simulink model "Overtaking"  (R2024a)
settings: Solver=FixedStepDiscrete  StartTime=0.0  StopTime=inf  FixedStep=0.001  RelTol=1e-3  EnableMultiTasking=on
undefined symbols (not defined in the file): route1_frenet, route1_waypoint, route2_frenet, route2_waypoint, route3_frenet, route3_waypoint, route4_frenet, route4_waypoint, route5_frenet, route5_waypoint
libraries: CarMaker4SL x49, simulink x1
(part 4 of 4)

== matlab function Overtaking/CarMaker/Subsystem/Final Project/Scenario 1/Waypoint_Follower1 ==
  settings: sampleTime=0.1
  data: local_waypoints input; steering_angle output; state input; change_dist input; target_idx output
% local tracking
function [steering_angle, target_idx] = waypoint_follower(local_waypoints, state, change_dist)

    WHEEL_BASE = 2.9;
    lookahead_dist = 6.0;
    
    % % sigmoid lookahead_dist change
    % if(change_dist > 1.8) 
    %     lookahead_dist = (10 / (1 + exp(-0.4 * change_dist))) + 5;
    % end
    % 
    % % final state -> parking area entry
    % if(state == 7)
    %     lookahead_dist = 2.5;
    % end

    target_idx = -1;
    final_ld = 0;

    for i = 1:size(local_waypoints, 1)
        dist = norm(local_waypoints(i, :));
        if dist > lookahead_dist && local_waypoints(i, 1) > 0
            target_idx = i;
            final_ld = dist;
            break;
        end
    end

    if target_idx == -1
        steering_angle = 0;
        return;
    end

    target_point = local_waypoints(target_idx, :);
    alpha = atan2(target_point(2), target_point(1));
    alpha = wrapToPi(alpha);

    final_ld = min(max(final_ld, 2.0), 20.0); 

    steering_angle = atan2(2 * WHEEL_BASE * sin(alpha), final_ld);
end


% % global tracking
% function [steering_angle, start_idx] = pure_pursuit(waypoints, vehicle_position, head)
% 
%     persistent last_target_idx;
%     if isempty(last_target_idx)
%         last_target_idx = 1; % 초기값 설정
%     end
% 
%     WHEEL_BASE = 2.7;
% 
%     waypoints_x = waypoints(:,1);
%     waypoints_y = waypoints(:,2);
%     % num_points = length(waypoints_x);
%     num_points = 300;
% 
%     local_waypoints = zeros(num_points, 2);
%     x_ego = vehicle_position(1);
%     y_ego = vehicle_position(2);
% 
%     for i = 1:num_points
%         dx = waypoints_x(i) - x_ego;
%         dy = waypoints_y(i) - y_ego;
% 
%         local_x = dx * cos(-head) - dy * sin(-head);
%         local_y = dx * sin(-head) + dy * cos(-head);
% 
%         local_waypoints(i, :) = [local_x, local_y];
%     end    
% 
%     lookahead_dist = 5.0;
% 
%     distances_to_waypoints = sqrt((waypoints_x - x_ego).^2 + (waypoints_y - y_ego).^2);
%     [~, closest_idx] = min(distances_to_waypoints);
% 
%     start_idx = max(last_target_idx, closest_idx);
% 
%     target_idx = -1;
%     final_ld = 0;
%     for i = start_idx:num_points
%         dist = norm(local_waypoints(i, :));
%         if dist > lookahead_dist && local_waypoints(i, 1) > 0
%             target_idx = i;
%             final_ld = dist;
%             break;
%         end
%     end
% 
%     if target_idx == -1
%         for i = 1:start_idx-1
%             dist = norm(local_waypoints(i, :));
%             if dist > lookahead_dist && local_waypoints(i, 1) > 0
%                 target_idx = i;
%                 final_ld = dist;
%                 break;
%             end
%         end
%     end
% 
%     if target_idx == -1
%         steering_angle = 0;
%         return;
%     end
% 
%     target_point = local_waypoints(target_idx, :);
%     alpha = atan2(target_point(2), target_point(1));
%     alpha = wrapToPi(alpha);
% 
%     final_ld = min(max(final_ld, 2.0), 20.0);
% 
%     steering_angle = atan2(2 * WHEEL_BASE * sin(alpha), final_ld);
% 
%     last_target_idx = target_idx;
% end

== stateflow chart Overtaking/CarMaker/Subsystem/Day3/Chart ==
  (default) -> (junction 1)
  (junction 1) -> (junction 3) [order 1] : [i<99]
      | {i = i + 1;}
  (junction 1) -> (junction 7) [order 2] : {i=0;}
  (junction 3) -> (junction 5)
  (junction 5) -> (junction 7)
  (junction 7) -> (junction 10)
  (junction 10) -> (junction 12) [order 1] : [rem(i,50) == 0]
      | {do_Logic;}
  (junction 10) -> (junction 18) [order 2]
  (junction 12) -> (junction 16)
  (junction 16) -> (junction 18)
  (junction 18) -> (junction 21)
  data: i local =0
  events: do_Logic output FUNCTION_CALL_EVENT
